simulink model "QAM_vold"  (R2015a)
settings: Solver=ode45  SolverMode=SingleTasking  StartTime=0.0  StopTime=0.1  FixedStep=10e-6  RelTol=10e-3
libraries: dspsrcs4 x4, commrandsrc2 x1, commdigbbndam3 x1
settings Model: CovMetricSettings=dwe  CovHtmlReporting=off  covSaveCumulativeToWorkspaceVar=off  CovSaveSingleToWorkspaceVar=off  CovExternalEMLEnable=on  Creator=marcone  LastModifiedBy=marcone
settings DataIOCC: LimitDataPoints=off  SaveFormat=Dataset
settings DebuggingCC: SFUnexpectedBacktrackingDiag=error  SFNoUnconditionalDefaultTransitionDiag=error
settings HardwareCC: ProdBitPerPointer=64  ProdLargestAtomicFloat=Float  ProdIntDivRoundTo=Zero  ProdEndianess=LittleEndian  ProdHWDeviceType=Specified
settings ModelReferenceCC: PropagateSignalLabelsOutOfModel=on
settings SFSimCC: SimUseLocalCustomCode=on
settings RTWCC: RTWUseLocalCustomCode=on
settings GRTTargetCC: TargetLangStandard=C99 (ISO)  GeneratePreprocessorConditionals=Use local settings

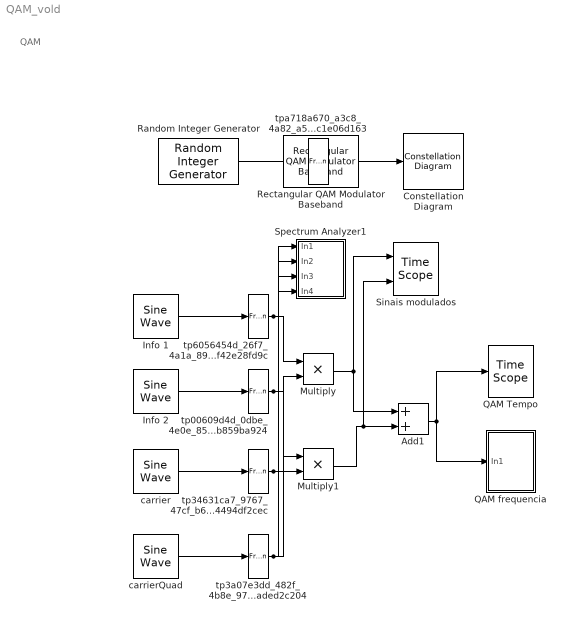
== system QAM_vold ==
  note: QAM
  Add1 : Sum
  Constellation Diagram : ConstellationDiagram
  Info 1 : dspsrcs4/Sine Wave  Amplitude=0.3  Frequency=2e3  Phase=0  SampleMode=Discrete  OutComplex=Real  CompMethod=Trigonometric fcn  TableSize=Speed  SampleTime=1/1e6  SamplesPerFrame=100  ResetState=Restart at time zero  dataType=double  wordLen=16  udDataType=sfix(16)  fracBitsMode=Best precision  numFracBits=15  OutDataTypeStr=double  LastOutDataTypeStr=double
  Info 2 : dspsrcs4/Sine Wave  Amplitude=0.5  Frequency=7e3  Phase=0  SampleMode=Discrete  OutComplex=Real  CompMethod=Trigonometric fcn  TableSize=Speed  SampleTime=1/1e6  SamplesPerFrame=100  ResetState=Restart at time zero  dataType=double  wordLen=16  udDataType=sfix(16)  fracBitsMode=Best precision  numFracBits=15  OutDataTypeStr=double  LastOutDataTypeStr=double
  Multiply : Product
  Multiply1 : Product
  QAM Tempo : TimeScope  DefaultConfigurationName=spbscopes.TimeScopeBlockCfg
  QAM frequencia : Subsystem  Description=Replaced Block  mask(Replaced Block){}
      mask help: This block has been replaced with an empty subsystem because it used functionality that is unavailable in Simulink R2015a.
      mask Display: fprintf('Replaced: %s\n','SpectrumAnalyzer')
  Random Integer Generator : commrandsrc2/Random Integer Generator  mul=4  seed=0  Ts=1  sampPerFrame=10000  outDataType=double  frameBased=on
  Rectangular QAM Modulator Baseband : commdigbbndam3/Rectangular QAM Modulator Baseband  M=4  InType=Integer  Enc=Gray  Mapping=[0:15]  PowType=Min. distance between symbols  MinDist=2  AvgPow=1  PeakPow=1  Ph=0  outDtype=double  outWordLen=16  outUDDataType=sfix(16)  outFracLenMode=Best precision  outFracLen=15
  Sinais modulados : TimeScope  DefaultConfigurationName=spbscopes.TimeScopeBlockCfg  NumInputPorts=2
  Spectrum Analyzer1 : Subsystem  Description=Replaced Block  mask(Replaced Block){}
      mask help: This block has been replaced with an empty subsystem because it used functionality that is unavailable in Simulink R2015a.
      mask Display: fprintf('Replaced: %s\n','SpectrumAnalyzer')
  carrier : dspsrcs4/Sine Wave  Amplitude=2  Frequency=100e3  Phase=0  SampleMode=Discrete  OutComplex=Real  CompMethod=Trigonometric fcn  TableSize=Speed  SampleTime=1/1e6  SamplesPerFrame=100  ResetState=Restart at time zero  dataType=double  wordLen=16  udDataType=sfix(16)  fracBitsMode=Best precision  numFracBits=15  OutDataTypeStr=double  LastOutDataTypeStr=double
  carrierQuad : dspsrcs4/Sine Wave  Amplitude=2  Frequency=100e3  Phase=90*pi/180  SampleMode=Discrete  OutComplex=Real  CompMethod=Trigonometric fcn  TableSize=Speed  SampleTime=1/1e6  SamplesPerFrame=100  ResetState=Restart at time zero  dataType=double  wordLen=16  udDataType=sfix(16)  fracBitsMode=Best precision  numFracBits=15  OutDataTypeStr=double  LastOutDataTypeStr=double
  tp00609d4d_0dbe_4e0e_8593_8c5b859ba924 : FrameConversion  OutFrame=Sample-based
  tp34631ca7_9767_47cf_b617_fd4494df2cec : FrameConversion  OutFrame=Sample-based
  tp3a07e3dd_482f_4b8e_975c_ed5aded2c204 : FrameConversion  OutFrame=Sample-based
  tp6056454d_26f7_4a1a_89de_27f42e28fd9c : FrameConversion  OutFrame=Sample-based
  tpa718a670_a3c8_4a82_a5e9_227c1e06d163 : FrameConversion  OutFrame=Sample-based
  wires:
  Multiply/1 -> Add1/1, Sinais modulados/1
  Multiply1/1 -> Sinais modulados/2, Add1/2
  Add1/1 -> QAM Tempo/1, QAM frequencia/1(In1)
  Rectangular QAM Modulator Baseband/1 -> Constellation Diagram/1
  Info 1/1 -> tp6056454d_26f7_4a1a_89de_27f42e28fd9c/1
  tp6056454d_26f7_4a1a_89de_27f42e28fd9c/1 -> Multiply/1, Spectrum Analyzer1/1(In1)
  Info 2/1 -> tp00609d4d_0dbe_4e0e_8593_8c5b859ba924/1
  tp00609d4d_0dbe_4e0e_8593_8c5b859ba924/1 -> Multiply1/1, Spectrum Analyzer1/2(In2)
  carrier/1 -> tp34631ca7_9767_47cf_b617_fd4494df2cec/1
  tp34631ca7_9767_47cf_b617_fd4494df2cec/1 -> Multiply/2, Spectrum Analyzer1/3(In3)
  carrierQuad/1 -> tp3a07e3dd_482f_4b8e_975c_ed5aded2c204/1
  tp3a07e3dd_482f_4b8e_975c_ed5aded2c204/1 -> Spectrum Analyzer1/4(In4), Multiply1/2
  Random Integer Generator/1 -> tpa718a670_a3c8_4a82_a5e9_227c1e06d163/1
  tpa718a670_a3c8_4a82_a5e9_227c1e06d163/1 -> Rectangular QAM Modulator Baseband/1

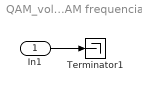
== system QAM_vold/QAM frequencia ==
  In1 : Inport
  Terminator1 : Terminator
  wires:
  In1/1 -> Terminator1/1

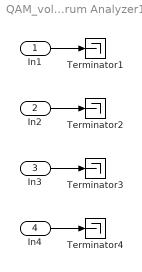
== system QAM_vold/Spectrum Analyzer1 ==
  In1 : Inport
  In2 : Inport  Port=2
  In3 : Inport  Port=3
  In4 : Inport  Port=4
  Terminator{1..4} (4 alike) : Terminator
  wires:
  In4/1 -> Terminator4/1
  In3/1 -> Terminator3/1
  In2/1 -> Terminator2/1
  In1/1 -> Terminator1/1
